simulink model "PDS"  (R2020a)
settings: Solver=VariableStepAuto  StartTime=0.0  StopTime=10.0  RelTol=1e-3
settings Model: Creator=HP  LastModifiedBy=HP

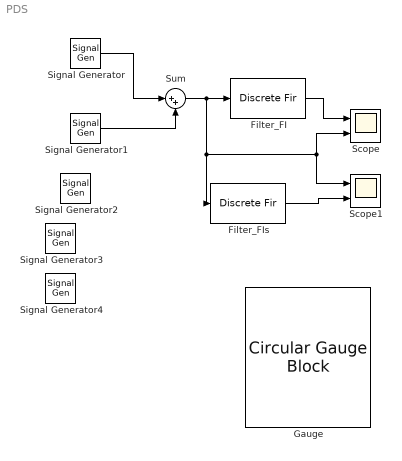
== system PDS ==
  Filter_FI : DiscreteFir  Tag=BlockMethodSubSystem  Coefficients=[0.00357339134833414319 0.00664771989932296317 0.0153299607846750941 0.0294048295549019095 0.0466563167060366144 0.0633940391432614853 0.0755543491619573571 0.0800000000000000017 0.0755543491619573571 0.0633940391432614853 0.0466563167060366144 0.0294048295549019095 0.0153299607846750941 0.00664771989932296317 0.00357339134833414319]  InputProcessing=Columns as channels (frame based)
  Filter_FIs : DiscreteFir  Tag=BlockMethodSubSystem  Coefficients=[0 -0.00572009152941761745 -0.0197901124196261831 -0.0340523480472841034 0.959999999999999964 -0.0340523480472841034 -0.0197901124196261831 -0.00572009152941761745 0]  InputProcessing=Columns as channels (frame based)
  Gauge : CircularGaugeBlock
  Scope : Scope  NumInputPorts=2
  Scope1 : Scope  NumInputPorts=2
  Signal Generator : SignalGenerator  Amplitude=2  Frequency=0.5
  Signal Generator{1..4} (4 alike) : SignalGenerator  Amplitude=0.2  Frequency=80  Units=rad/sec
  Sum : Sum  Inputs=|++
  wires:
  Signal Generator/1 -> Sum/1
  Signal Generator1/1 -> Sum/2
  Filter_FI/1 -> Scope/1
  Sum/1 -> Filter_FIs/1, Scope1/1, Scope/2, Filter_FI/1
  Filter_FIs/1 -> Scope1/2
